simulink model "humidifier"  (R2021a)
settings: Solver=VariableStepAuto  StartTime=0.0  StopTime=inf  FixedStep=100  MaxStep=1000.0  MinStep=500.0  RelTol=1e-3  EnableMultiTasking=on
model workspace (MAT data in the model file):
  H_tol = 3
  T_tol = 2
libraries: simulink x1
settings Model: ExtModeAutoUpdateStatusClock=off  Creator=The MathWorks, Inc.  LastModifiedBy=vlads
settings SolverCC: AlgebraicLoopSolver=TrustRegion
settings DataIOCC: LimitDataPoints=on  SaveFormat=Array  ReturnWorkspaceOutputs=off
settings OptimizationCC: ExpressionDepthLimit=2147483647  InitFltsAndDblsToZero=on  EfficientMapNaN2IntZero=off  LifeSpan=inf
settings DebuggingCC: SaveWithParameterizedLinksMsg=none  UnderspecifiedInitializationDetection=Classic  MergeDetectMultiDrivingBlocksExec=none  SignalResolutionControl=TryResolveAllWithWarning  SolverPrmCheckMsg=warning  MultiTaskDSMMsg=warning  MultiTaskCondExecSysMsg=none  FcnCallInpInsideContextMsg=warning  StateNameClashWarn=warning  SFUnexpectedBacktrackingDiag=warning  SFNoUnconditionalDefaultTransitionDiag=warning  SFExecutionAtInitializationDiag=none  SFMachineParentedDataDiag=warning  ArithmeticOperatorsInVariantConditions=warning
settings HardwareCC: ProdBitPerPointer=32  ProdBitPerSizeT=32  ProdBitPerPtrDiffT=32  ProdLargestAtomicFloat=None  ProdIntDivRoundTo=Undefined  ProdEndianess=Unspecified  ProdWordSize=32  ProdHWDeviceType=32-bit Generic
settings ModelReferenceCC: PropagateSignalLabelsOutOfModel=off
settings SFSimCC: SimUseLocalCustomCode=off  SimParseCustomCode=off  CustomCodeUndefinedFunction=UseInterfaceOnly
settings RTWCC: RTWUseLocalCustomCode=off
settings CodeAppCC: StateflowObjectComments=on
settings GRTTargetCC: TargetFcnLib=ansi_tfl_tmw.mat  TargetLangStandard=C89/C90 (ANSI)  CombineOutputUpdateFcns=off  GRTInterface=on
settings ConfigComp: CovMetricSettings=dw  CovSaveCumulativeToWorkspaceVar=on  CovSaveSingleToWorkspaceVar=on  CovExternalEMLEnable=off  CovSFcnEnable=off

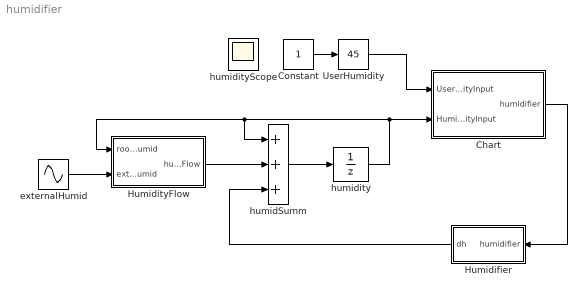
== system humidifier ==
  Chart : Stateflow chart  TreatAsAtomicUnit=on
  Constant : Constant
  Humidifier : Subsystem  TreatAsAtomicUnit=on
  HumidityFlow : Subsystem  TreatAsAtomicUnit=on
  UserHumidity : simulink/Math Operations/Slider Gain  gain=45  low=0  high=100
  externalHumid : Sin  SineType=Sample based  Amplitude=10  Bias=45  Frequency=1/(24*60)  Samples=2500  SampleTime=1
  humidSumm : Sum  Inputs=+++  RndMeth=Zero
  humidity : UnitDelay  InitialCondition=45  HasFrameUpgradeWarning=on
  humidityScope : Scope
      settings: Floating=on
  wires:
  Humidifier/1(dh) -> humidSumm/3
  externalHumid/1 -> HumidityFlow/2(externalHumid)
  humidSumm/1 -> humidity/1
  humidity/1 -> Chart/2(HumidityInput), HumidityFlow/1(roomHumid), humidSumm/1
  HumidityFlow/1(humidFlow) -> humidSumm/2
  Constant/1 -> UserHumidity/1
  UserHumidity/1 -> Chart/1(UserHumidityInput)
  Chart/1(humidifier) -> Humidifier/1(humidifier)

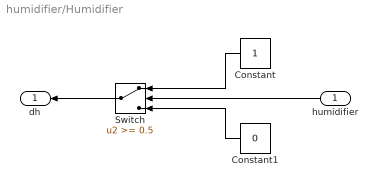
== system humidifier/Humidifier ==
  humidifier : Inport
  Constant : Constant
  Constant1 : Constant  Value=0
  Switch : Switch  Threshold=0.5
  dh : Outport  OutDataTypeStr=double  InitialOutput=0  VectorParamsAs1DForOutWhenUnconnected=off
  wires:
  humidifier/1 -> Switch/2
  Constant/1 -> Switch/1
  Constant1/1 -> Switch/3
  Switch/1 -> dh/1

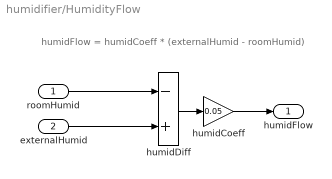
== system humidifier/HumidityFlow ==
  note: humidFlow = humidCoeff * (externalHumid - roomHumid)
  roomHumid : Inport
  externalHumid : Inport  Port=2
  humidCoeff : Gain  Gain=0.05
  humidDiff : Sum  Inputs=-+
  humidFlow : Outport  OutDataTypeStr=double  InitialOutput=0  VectorParamsAs1DForOutWhenUnconnected=off
  wires:
  humidCoeff/1 -> humidFlow/1
  humidDiff/1 -> humidCoeff/1
  roomHumid/1 -> humidDiff/1
  externalHumid/1 -> humidDiff/2

== stateflow chart humidifier/Chart ==
  state CheckHumidity
    Humidity = HumidityInput;
    UserHumidity = UserHumidityInput;
  state HumidifierOn
    humidifier = 1;
  state HumidifierOff
    humidifier = 0;
  (default) -> CheckHumidity
  HumidifierOn -> CheckHumidity : {after(5, sec)}
  HumidifierOff -> CheckHumidity : {after(5, sec)
      | }
  CheckHumidity -> HumidifierOn [order 1] : [Humidity < UserHumidity]
  CheckHumidity -> HumidifierOff [order 2] : [Humidity >= UserHumidity]
  data: UserHumidityInput input; HumidityInput input; humidifier output; UserHumidity local; Humidity local
